simulink model "loadOperator"  (Simulink 8.1)
settings: Solver=ode45  StartTime=0.0  StopTime=inf  RelTol=1e-3
settings Model: Creator=eiseles  LastModifiedBy=eiseles
settings DataIOCC: SignalLoggingSaveFormat=Dataset
settings OptimizationCC: ExpressionDepthLimit=128
settings DebuggingCC: FcnCallInpInsideContextMsg=EnableAllAsError
settings GRTTargetCC: CombineOutputUpdateFcns=on  GRTInterface=off

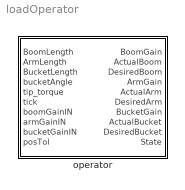
== system loadOperator ==
  operator : Subsystem

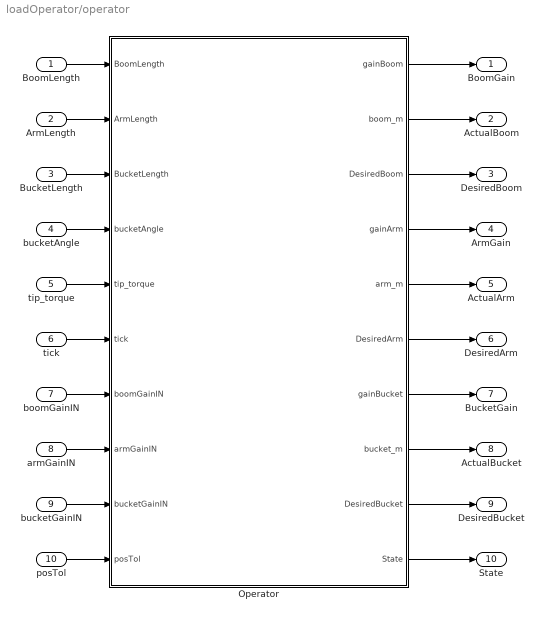
== system loadOperator/operator ==
  BoomLength : Inport
  ArmLength : Inport  Port=2
  BucketLength : Inport  Port=3
  bucketAngle : Inport  Port=4
  tip_torque : Inport  Port=5
  tick : Inport  Port=6
  boomGainIN : Inport  Port=7
  armGainIN : Inport  Port=8
  bucketGainIN : Inport  Port=9
  posTol : Inport  Port=10
  Operator : Stateflow chart  TreatAsAtomicUnit=on
  BoomGain : Outport
  ActualBoom : Outport  Port=2
  DesiredBoom : Outport  Port=3
  ArmGain : Outport  Port=4
  ActualArm : Outport  Port=5
  DesiredArm : Outport  Port=6
  BucketGain : Outport  Port=7
  ActualBucket : Outport  Port=8
  DesiredBucket : Outport  Port=9
  State : Outport  Port=10
  wires:
  bucketAngle/1 -> Operator/4(bucketAngle)
  BoomLength/1 -> Operator/1(BoomLength)
  BucketLength/1 -> Operator/3(BucketLength)
  tip_torque/1 -> Operator/5(tip_torque)
  ArmLength/1 -> Operator/2(ArmLength)
  Operator/2(boom_m) -> ActualBoom/1
  Operator/3(DesiredBoom) -> DesiredBoom/1
  Operator/4(gainArm) -> ArmGain/1
  Operator/1(gainBoom) -> BoomGain/1
  Operator/6(DesiredArm) -> DesiredArm/1
  Operator/7(gainBucket) -> BucketGain/1
  Operator/9(DesiredBucket) -> DesiredBucket/1
  Operator/5(arm_m) -> ActualArm/1
  Operator/8(bucket_m) -> ActualBucket/1
  tick/1 -> Operator/6(tick)
  Operator/10(State) -> State/1
  boomGainIN/1 -> Operator/7(boomGainIN)
  armGainIN/1 -> Operator/8(armGainIN)
  bucketGainIN/1 -> Operator/9(bucketGainIN)
  posTol/1 -> Operator/10(posTol)

== stateflow chart operator/Operator ==
  state intial
    en: State = 0;
    DesiredBoom = BoomLength;
    DesiredArm = ArmLength;
    DesiredBucket = BucketLength;
    gainBoom = boomGainIN;
    gainArm = armGainIN;
    gainBucket = bucketGainIN;
    during:boom_m = BoomLength;
    arm_m = ArmLength;
    bucket_m = BucketLength;
  (default) -> intial
  data: gainBoom output double =1; boom_m output double; DesiredBoom output double; gainArm output double =1; arm_m output double; DesiredArm output double; BoomLength input double; ArmLength input double; BucketLength input double; bucketAngle input double; gainBucket output double =1; bucket_m output double; DesiredBucket output double; tip_torque input double; max_torque local double =1e5; tick input double; State output double; FinalArm local double; levelBucket local double =1.8; boomGainIN input double; armGainIN input double; bucketGainIN input double; posTol input double
